simulink model "kalmn"  (R2022a)
settings: Solver=VariableStepAuto  StartTime=0.0  StopTime=80  RelTol=1e-3
undefined symbols (not defined in the file or in its folder): A, C, D, Discrete, Time
libraries: ctrlSharedLib x1
settings Model: Creator=baswarajswamy  LastModifiedBy=baswarajswamy

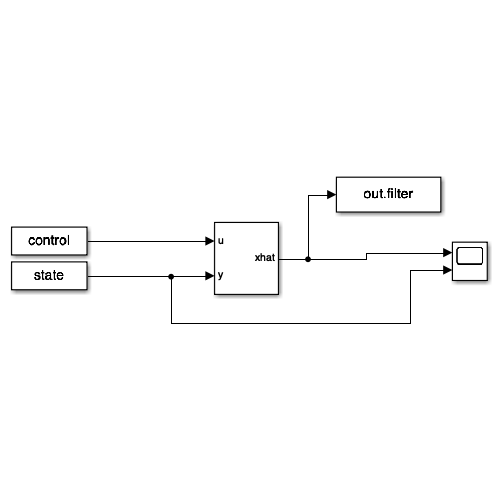
[thumbnail: Simulink's stored preview of the top-level diagram]
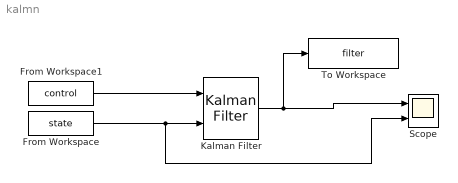
== system kalmn ==
  From Workspace : FromWorkspace  VariableName=state  SampleTime=0.2
  From Workspace1 : FromWorkspace  VariableName=control  SampleTime=0.2
  Kalman Filter : ctrlSharedLib/Kalman Filter  TimeDomain=Discrete-Time  UseCurrentEstimator=on  ModelSource=Individual A, B, C, D matrices  ModelSourceVariable=ss(0.95,1,1,0,1)  A=A  B=diag([0.2 0.2 0.2 0.2 0.2 0.2])  C=C  D=D  NumberOfStates=1  NumberOfInputs=1  NumberOfOutputs=1  InitialEstimateSource=Dialog  X0=0  P0=10  UseK=off  UseGH=off  NumberOfProcessNoiseInputs=1  G=1  TimeInvariantG=on  H=0  TimeInvariantH=on  Q=0.05  TimeInvariantQ=on  R=0.8  TimeInvariantR=on  N=0  TimeInvariantN=on  AddInputPort=on  AddEnablePort=off  OutputEstimatedY=off  OutputP=off  Ts=0.2
  Scope : Scope  NumInputPorts=2
  To Workspace : ToWorkspace  VariableName=filter  SaveFormat=Timeseries  SampleTime=-1
  wires:
  From Workspace/1 -> Scope/2, Kalman Filter/2
  From Workspace1/1 -> Kalman Filter/1
  Kalman Filter/1 -> To Workspace/1, Scope/1
